simulink model "main_acs_sitl"  (R2025b)
settings: Solver=VariableStepAuto  StartTime=0.0  StopTime=20  RelTol=1e-3
libraries: instrumentlib x2
settings Model: Creator=Filip  LastModifiedBy=Filip

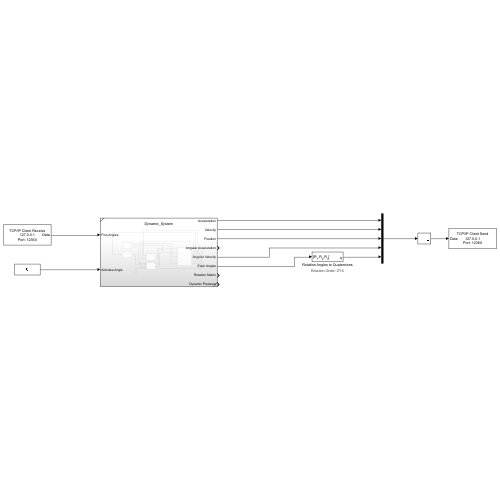
[thumbnail: Simulink's stored preview of the top-level diagram]
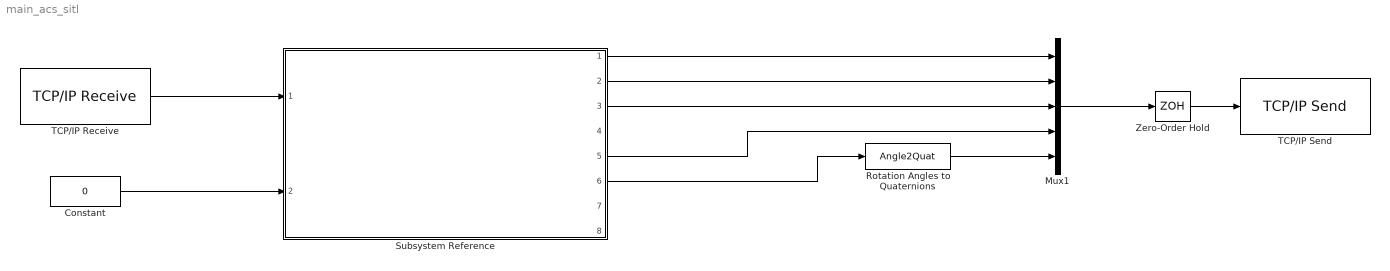
== system main_acs_sitl ==
  Constant : Constant  Value=0
  Mux1 : Mux  Inputs=5
  Rotation Angles to Quaternions : Angle2Quat
      settings: AttributesFormatString=Rotation Order: %<rotationOrder>
  Subsystem Reference : Subsystem  ReferencedSubsystem=Dynamic_System
  TCP/IP Receive : instrumentlib/TCP//IP Receive  Host=127.0.0.1  Port=12360  DataSize=[ 4, 1 ]  DataType=double  ASCIIFormatting=%f  Terminator=LF  CustomTerminator=10  ByteOrder=little-endian  EnableBlockingMode=on  Timeout=10  SampleTime=0.001  SimulateUsing=Interpreted execution
  TCP/IP Send : instrumentlib/TCP//IP Send  Host=127.0.0.1  Port=12360  ByteOrder=little-endian  EnableBlockingMode=on  Timeout=10  TransferDelay=off  SimulateUsing=Interpreted execution
  Zero-Order Hold : ZeroOrderHold  SampleTime=0.001
  wires:
  TCP/IP Receive/1 -> Subsystem Reference/1
  Zero-Order Hold/1 -> TCP/IP Send/1
  Subsystem Reference/3 -> Mux1/3
  Subsystem Reference/6 -> Rotation Angles to Quaternions/1
  Subsystem Reference/2 -> Mux1/2
  Subsystem Reference/1 -> Mux1/1
  Rotation Angles to Quaternions/1 -> Mux1/5
  Subsystem Reference/5 -> Mux1/4
  Mux1/1 -> Zero-Order Hold/1
  Constant/1 -> Subsystem Reference/2
